simulink model "ASW_PhCurrGen"  (R2023a)
settings: configuration reference "cfg_FastTaskCodeGeneration_v01" (kept outside this file)
undefined symbols (not defined in the file): Cdbl_tiSlwTaskSmpTi, Gu16_psiPermMagFlx_C
settings Model: DataDictionary=dd_foc_dictionary.sldd  EnableAccessToBaseWorkspace=off  Creator=WFYXQ  LastModifiedBy=xiaoqiang.yuan
settings ConfigSetRef: SourceName=cfg_FastTaskCodeGeneration_v01

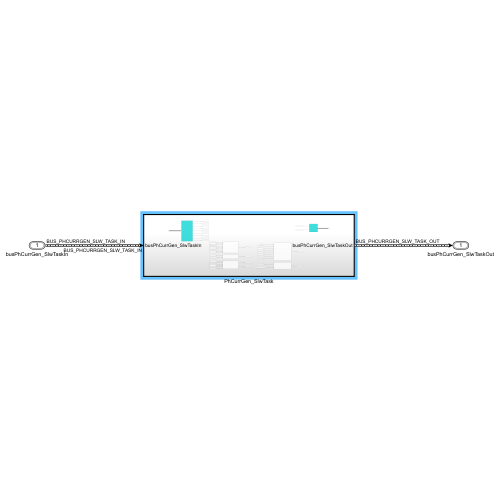
[thumbnail: Simulink's stored preview of the top-level diagram]
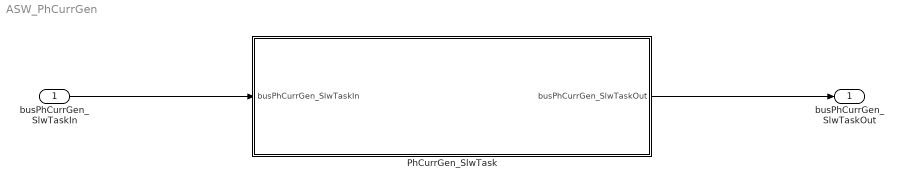
== system ASW_PhCurrGen ==
  busPhCurrGen_SlwTaskIn : Inport  OutDataTypeStr=Bus: BUS_PHCURRGEN_SLW_TASK_IN  SampleTime=round(double(Cdbl_tiSlwTaskSmpTi),4)  BusOutputAsStruct=on
  PhCurrGen_SlwTask : Subsystem  TreatAsAtomicUnit=on  RTWFcnName=PhCurrGen_SlwTask
      settings: RTWSystemCode=Nonreusable function  RTWFcnNameOpts=User specified
  busPhCurrGen_SlwTaskOut : Outport  OutDataTypeStr=Bus: BUS_PHCURRGEN_SLW_TASK_OUT  SampleTime=round(double(Cdbl_tiSlwTaskSmpTi),4)
  wires:
  busPhCurrGen_SlwTaskIn/1 -> PhCurrGen_SlwTask/1(busPhCurrGen_SlwTaskIn)
  PhCurrGen_SlwTask/1(busPhCurrGen_SlwTaskOut) -> busPhCurrGen_SlwTaskOut/1

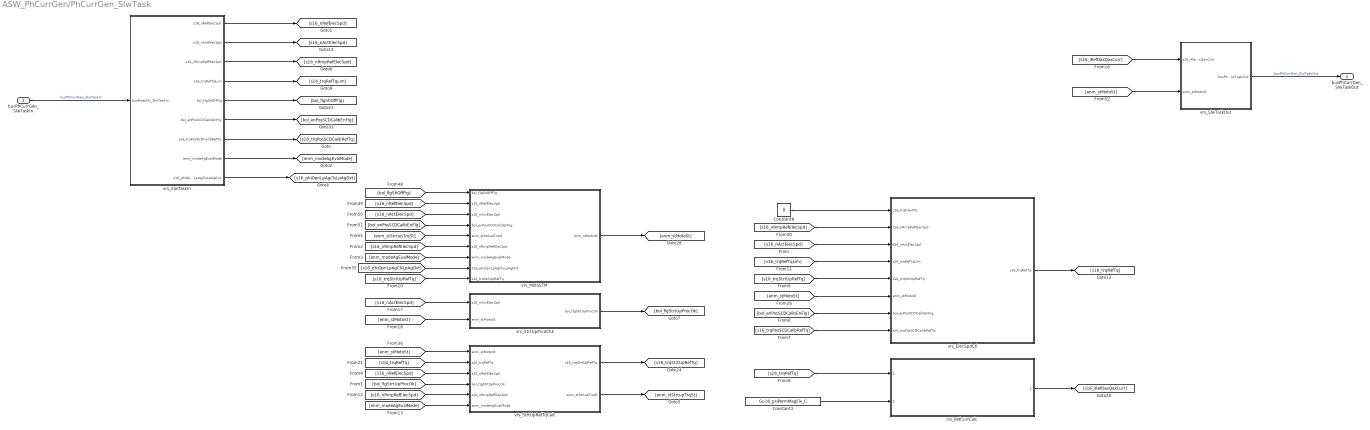
== system ASW_PhCurrGen/PhCurrGen_SlwTask ==
  busPhCurrGen_SlwTaskIn : Inport
  Constant3 : Constant  Value=Gu16_psiPermMagFlx_C
  Constant8 : Constant  Value=0  OutDataTypeStr=dt_Standardize_s16p15b0
  rss_RefCurrCalc : Subsystem  ReferencedSubsystem=rss_RefCurrCalc
  vrs_ElecSpdCtl : Subsystem  Variant=on  VariantControlMode=label  VariantControl=Choice  LabelModeActiveChoice=cstHybrCtrlLbl
  vrs_MotoSTM : Subsystem  Variant=on  VariantControlMode=label  LabelModeActiveChoice=cstHybrCtrlLbl
  vrs_SlwTaskIn : Subsystem  Variant=on  VariantControlMode=label  VariantControl=cstSenlCtrlLbl  LabelModeActiveChoice=cstHybrCtrlLbl
  vrs_SlwTaskOut : Subsystem  Variant=on  VariantControlMode=label  VariantControl=Choice  LabelModeActiveChoice=cstSenlCtrlLbl
  vrs_StrtUpPrcdChk : Subsystem  Variant=on  VariantControlMode=label  LabelModeActiveChoice=cstSenlCtrlLbl
  vrs_StrtUpRefTqCalc : Subsystem  Variant=on  VariantControlMode=label  LabelModeActiveChoice=cstSenlCtrlLbl
  busPhCurrGen_SlwTaskOut : Outport
  wires:
  [s16_trqRefTqLim] -> vrs_ElecSpdCtl/4(s16_trqRefTqLim)
  [s16_iRefDaxQaxCurr] -> vrs_SlwTaskOut/1(s16_iRefDaxQaxCurr)
  Constant8/1 -> vrs_ElecSpdCtl/1(s16_trqFdwdTq)
  vrs_SlwTaskOut/1(busPhCurrGen_SlwTaskOut) -> busPhCurrGen_SlwTaskOut/1  "busPhCurrGen_SlwTaskOut"
  vrs_StrtUpPrcdChk/1(bol_flgStrtUpProcOk) -> [bol_flgStrtUpProcOk]
  [enm_stMotoSt] -> vrs_StrtUpPrcdChk/2(enm_stMotoSt)
  [s16_trqRefTq] -> rss_RefCurrCalc/1
  vrs_ElecSpdCtl/1(s16_trqRefTq) -> [s16_trqRefTq]
  rss_RefCurrCalc/1 -> [s16_iRefDaxQaxCurr]
  [s16_nRmpRefElecSpd] -> vrs_ElecSpdCtl/2(s16_nRmpRefElecSpd)
  [s16_nActElecSpd] -> vrs_StrtUpPrcdChk/1(s16_nActElecSpd)
  [s16_nActElecSpd] -> vrs_ElecSpdCtl/3(s16_nActElecSpd)
  [enm_stMotoSt] -> vrs_ElecSpdCtl/6(enm_stMotoSt)
  [bol_flgShOffFlg] -> vrs_MotoSTM/1(bol_flgShOffFlg)
  [s16_nRefElecSpd] -> vrs_MotoSTM/2(s16_nRefElecSpd)
  [s16_nActElecSpd] -> vrs_MotoSTM/3(s16_nActElecSpd)
  [bol_enPosSCDCalibEnFlg] -> vrs_MotoSTM/4(bol_enPosSCDCalibEnFlg)
  vrs_MotoSTM/1(enm_stMotoSt) -> [enm_stMotoSt]
  [enm_stMotoSt] -> vrs_SlwTaskOut/2(enm_stMotoSt)
  [bol_enPosSCDCalibEnFlg] -> vrs_ElecSpdCtl/7(bol_enPosSCDCalibEnFlg)
  [s16_trqPosSCDCalibRefTq] -> vrs_ElecSpdCtl/8(s16_trqPosSCDCalibRefTq)
  [s16_trqStrtUpRefTq] -> vrs_ElecSpdCtl/5(s16_trqStrtUpRefTq)
  [enm_stMotoSt] -> vrs_StrtUpRefTqCalc/1(enm_stMotoSt)
  [s16_trqRefTq] -> vrs_StrtUpRefTqCalc/2(s16_trqRefTq)
  vrs_StrtUpRefTqCalc/1(s16_trqStrtUpRefTq) -> [s16_trqStrtUpRefTq]
  [s16_nRmpRefElecSpd] -> vrs_MotoSTM/6(s16_nRmpRefElecSpd)
  busPhCurrGen_SlwTaskIn/1 -> vrs_SlwTaskIn/1(busMotoCtl_SlwTaskIn)  "busPhCurrGen_SlwTaskIn"
  vrs_SlwTaskIn/1(s16_nRefElecSpd) -> [s16_nRefElecSpd]
  vrs_SlwTaskIn/2(s16_nActElecSpd) -> [s16_nActElecSpd]
  vrs_SlwTaskIn/3(s16_nRmpRefElecSpd) -> [s16_nRmpRefElecSpd]
  vrs_SlwTaskIn/4(s16_trqRefTqLim) -> [s16_trqRefTqLim]
  vrs_SlwTaskIn/5(bol_flgShOffFlg) -> [bol_flgShOffFlg]
  vrs_SlwTaskIn/6(bol_enPosSCDCalibEnFlg) -> [bol_enPosSCDCalibEnFlg]
  vrs_SlwTaskIn/7(s16_trqPosSCDCalibRefTq) -> [s16_trqPosSCDCalibRefTq]
  vrs_SlwTaskIn/8(enm_modeAgEvalMode) -> [enm_modeAgEvalMode]
  [enm_modeAgEvalMode] -> vrs_MotoSTM/7(enm_modeAgEvalMode)
  Constant3/1 -> rss_RefCurrCalc/2
  [s16_nRefElecSpd] -> vrs_StrtUpRefTqCalc/3(s16_nRefElecSpd)
  vrs_StrtUpRefTqCalc/2(enm_stStrtupTrqSt) -> [enm_stStrtupTrqSt]
  [bol_flgStrtUpProcOk] -> vrs_StrtUpRefTqCalc/4(bol_flgStrtUpProcOk)
  [s16_nRmpRefElecSpd] -> vrs_StrtUpRefTqCalc/5(s16_nRmpRefElecSpd)
  [enm_modeAgEvalMode] -> vrs_StrtUpRefTqCalc/6(enm_modeAgEvalMode)
  [enm_stStrtupTrqSt] -> vrs_MotoSTM/5(enm_stStrtupTrqSt)
  [s16_phiOpnLpAgClsLpAgDvt] -> vrs_MotoSTM/8(s16_phiOpnLpAgClsLpAgDvt)
  [s16_trqStrtUpRefTq] -> vrs_MotoSTM/9(s16_trqStrtUpRefTq)
  vrs_SlwTaskIn/9(s16_phiOpnLpAgClsLpAgDvt) -> [s16_phiOpnLpAgClsLpAgDvt]

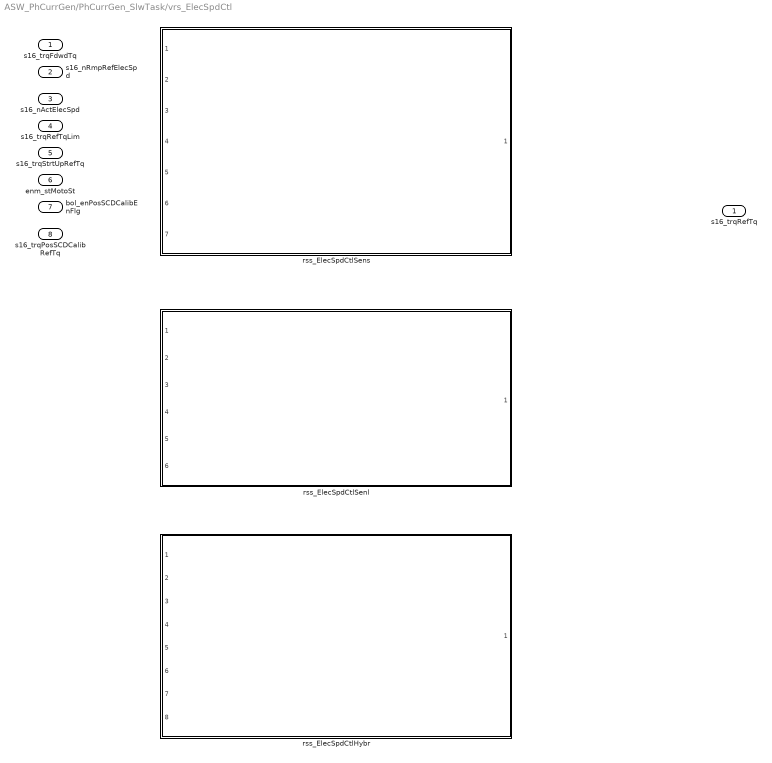
== system ASW_PhCurrGen/PhCurrGen_SlwTask/vrs_ElecSpdCtl ==
  s16_trqFdwdTq : Inport
  s16_nRmpRefElecSpd : Inport  Port=2
  s16_nActElecSpd : Inport  Port=3
  s16_trqRefTqLim : Inport  Port=4
  s16_trqStrtUpRefTq : Inport  Port=5
  enm_stMotoSt : Inport  Port=6
  bol_enPosSCDCalibEnFlg : Inport  Port=7
  s16_trqPosSCDCalibRefTq : Inport  Port=8
  rss_ElecSpdCtlHybr : Subsystem  VariantControl=cstHybrCtrlLbl  ReferencedSubsystem=rss_ElecSpdCtlHybr
  rss_ElecSpdCtlSenl : Subsystem  VariantControl=cstSenlCtrlLbl  ReferencedSubsystem=rss_ElecSpdCtlSenl
  rss_ElecSpdCtlSens : Subsystem  VariantControl=cstSensCtrlLbl  ReferencedSubsystem=rss_ElecSpdCtlSens
  s16_trqRefTq : Outport

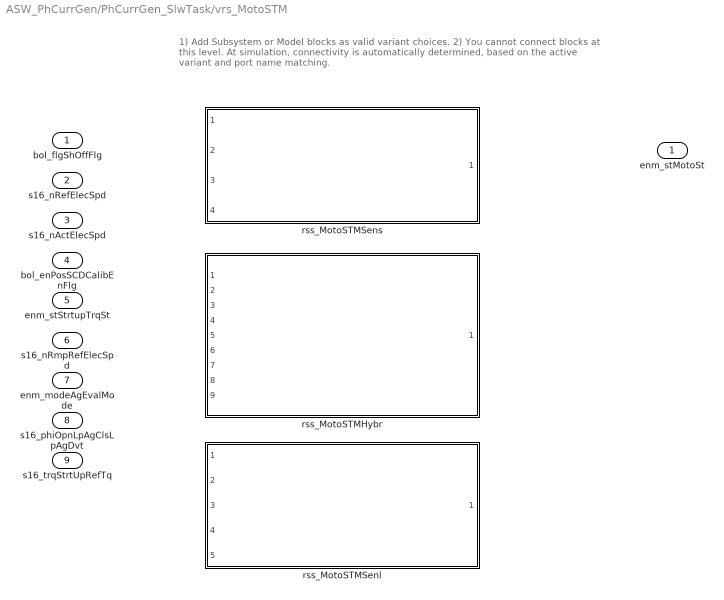
== system ASW_PhCurrGen/PhCurrGen_SlwTask/vrs_MotoSTM ==
  note: 1) Add Subsystem or Model blocks as valid variant choices.
      | 2) You cannot connect blocks at this level. At simulation, connectivity is automatically
      | determined, based on the active variant and port name matching.
  bol_flgShOffFlg : Inport
  s16_nRefElecSpd : Inport  Port=2
  s16_nActElecSpd : Inport  Port=3
  bol_enPosSCDCalibEnFlg : Inport  Port=4
  enm_stStrtupTrqSt : Inport  Port=5
  s16_nRmpRefElecSpd : Inport  Port=6
  enm_modeAgEvalMode : Inport  Port=7
  s16_phiOpnLpAgClsLpAgDvt : Inport  Port=8
  s16_trqStrtUpRefTq : Inport  Port=9
  rss_MotoSTMHybr : Subsystem  VariantControl=cstHybrCtrlLbl  ReferencedSubsystem=rss_MotoSTMHybr
  rss_MotoSTMSenl : Subsystem  VariantControl=cstSenlCtrlLbl  ReferencedSubsystem=rss_MotoSTMSenl
  rss_MotoSTMSens : Subsystem  VariantControl=cstSensCtrlLbl  ReferencedSubsystem=rss_MotoSTMSens
  enm_stMotoSt : Outport

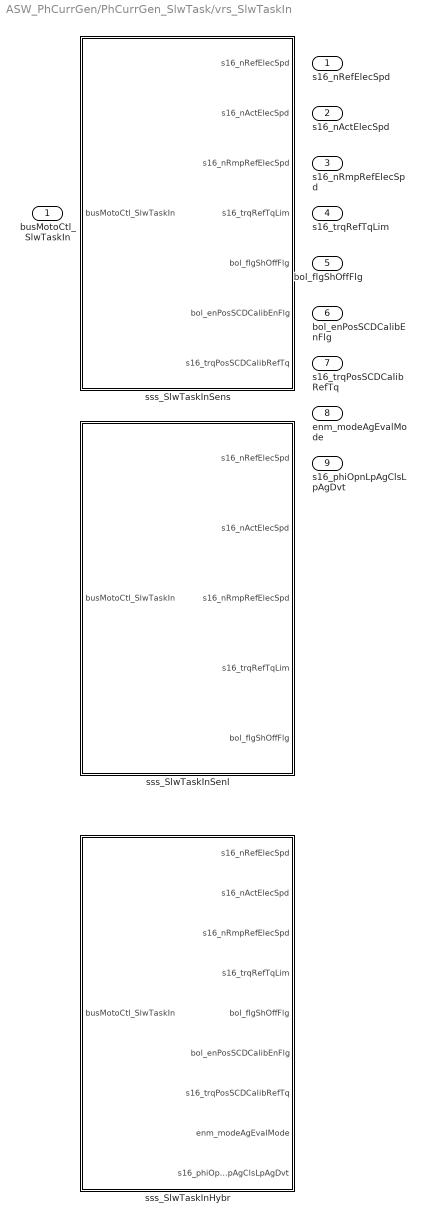
== system ASW_PhCurrGen/PhCurrGen_SlwTask/vrs_SlwTaskIn ==
  busMotoCtl_SlwTaskIn : Inport
  sss_SlwTaskInHybr : Subsystem  VariantControl=cstHybrCtrlLbl
  sss_SlwTaskInSenl : Subsystem  VariantControl=cstSenlCtrlLbl
  sss_SlwTaskInSens : Subsystem  VariantControl=cstSensCtrlLbl
  s16_nRefElecSpd : Outport
  s16_nActElecSpd : Outport  Port=2
  s16_nRmpRefElecSpd : Outport  Port=3
  s16_trqRefTqLim : Outport  Port=4
  bol_flgShOffFlg : Outport  Port=5
  bol_enPosSCDCalibEnFlg : Outport  Port=6
  s16_trqPosSCDCalibRefTq : Outport  Port=7
  enm_modeAgEvalMode : Outport  Port=8
  s16_phiOpnLpAgClsLpAgDvt : Outport  Port=9

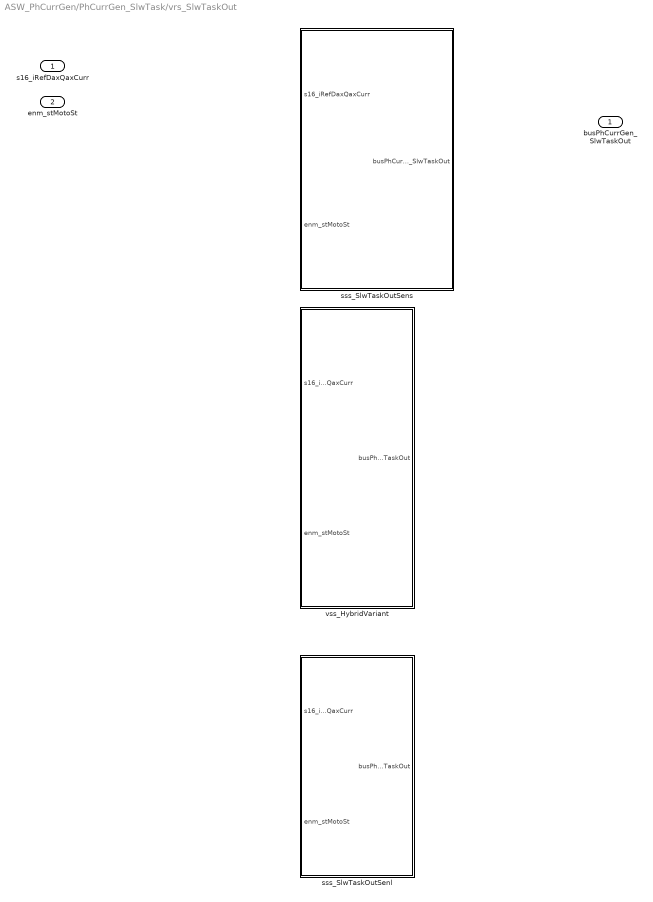
== system ASW_PhCurrGen/PhCurrGen_SlwTask/vrs_SlwTaskOut ==
  s16_iRefDaxQaxCurr : Inport
  enm_stMotoSt : Inport  Port=2
  sss_SlwTaskOutSenl : Subsystem  VariantControl=cstSenlCtrlLbl
  sss_SlwTaskOutSens : Subsystem  VariantControl=cstSensCtrlLbl
  vss_HybridVariant : Subsystem  VariantControl=cstHybrCtrlLbl
  busPhCurrGen_SlwTaskOut : Outport

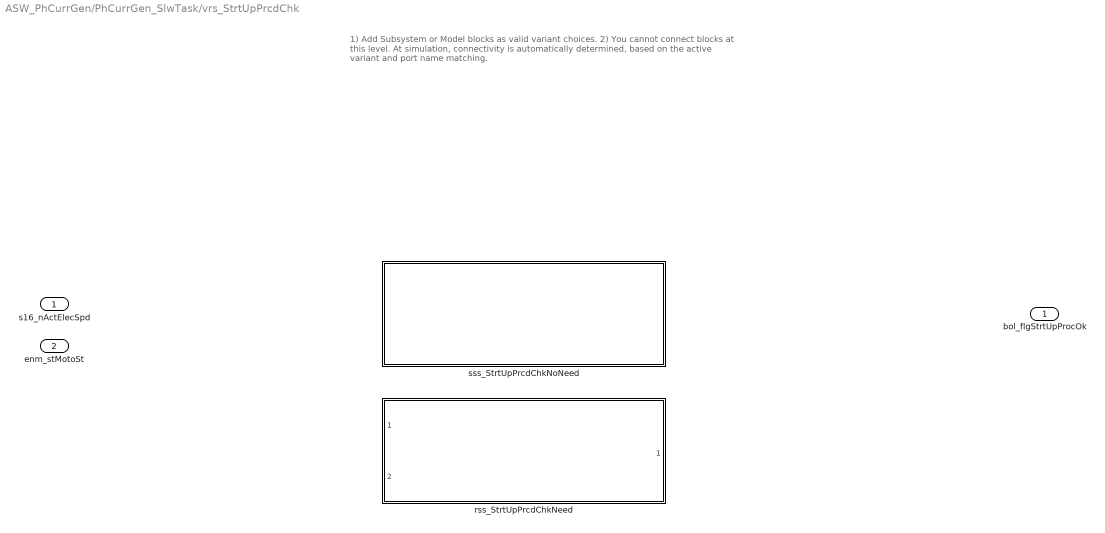
== system ASW_PhCurrGen/PhCurrGen_SlwTask/vrs_StrtUpPrcdChk ==
  note: 1) Add Subsystem or Model blocks as valid variant choices.
      | 2) You cannot connect blocks at this level. At simulation, connectivity is automatically
      | determined, based on the active variant and port name matching.
  s16_nActElecSpd : Inport  PortDimensions=1
  enm_stMotoSt : Inport  Port=2
  rss_StrtUpPrcdChkNeed : Subsystem  VariantControl=cstSenlCtrlLbl  ReferencedSubsystem=rss_StrtUpPrcdChkNeed
  sss_StrtUpPrcdChkNoNeed : Subsystem  VariantControl=cstSensCtrlLbl
  bol_flgStrtUpProcOk : Outport

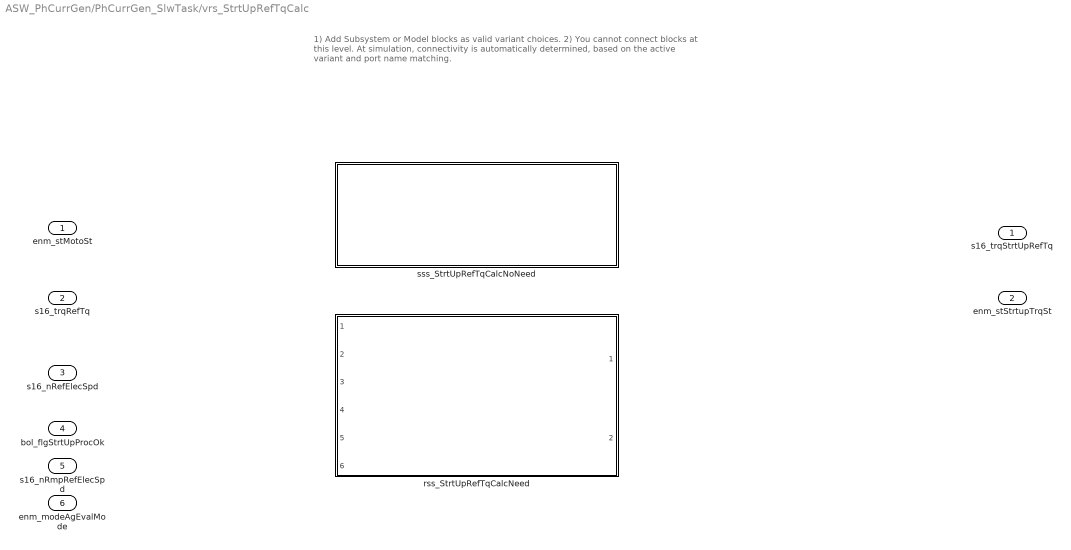
== system ASW_PhCurrGen/PhCurrGen_SlwTask/vrs_StrtUpRefTqCalc ==
  note: 1) Add Subsystem or Model blocks as valid variant choices.
      | 2) You cannot connect blocks at this level. At simulation, connectivity is automatically
      | determined, based on the active variant and port name matching.
  enm_stMotoSt : Inport
  s16_trqRefTq : Inport  Port=2
  s16_nRefElecSpd : Inport  Port=3
  bol_flgStrtUpProcOk : Inport  Port=4
  s16_nRmpRefElecSpd : Inport  Port=5
  enm_modeAgEvalMode : Inport  Port=6
  rss_StrtUpRefTqCalcNeed : Subsystem  VariantControl=cstSenlCtrlLbl  ReferencedSubsystem=rss_StrtUpRefTqCalcNeed
  sss_StrtUpRefTqCalcNoNeed : Subsystem  VariantControl=cstSensCtrlLbl
  s16_trqStrtUpRefTq : Outport
  enm_stStrtupTrqSt : Outport  Port=2

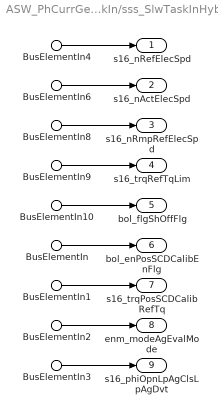
== system ASW_PhCurrGen/PhCurrGen_SlwTask/vrs_SlwTaskIn/sss_SlwTaskInHybr ==
  BusElementIn4 : Inport  PortName=busMotoCtl_SlwTaskIn  Element=s16_nRefElecSpd
  BusElementIn6 : Inport  PortName=busMotoCtl_SlwTaskIn  Element=s16_nActElecSpd
  BusElementIn8 : Inport  PortName=busMotoCtl_SlwTaskIn  Element=s16_nRmpRefElecSpd
  BusElementIn9 : Inport  PortName=busMotoCtl_SlwTaskIn  Element=s16_trqRefTqLim
  BusElementIn10 : Inport  PortName=busMotoCtl_SlwTaskIn  Element=bol_flgShOffFlg
  BusElementIn : Inport  PortName=busMotoCtl_SlwTaskIn  Element=bol_enPosSCDCalibEnFlg
  BusElementIn1 : Inport  PortName=busMotoCtl_SlwTaskIn  Element=s16_trqPosSCDCalibRefTq
  BusElementIn2 : Inport  PortName=busMotoCtl_SlwTaskIn  Element=enm_modeAgEvalMode
  BusElementIn3 : Inport  PortName=busMotoCtl_SlwTaskIn  Element=s16_phiOpnLpAgClsLpAgDvt
  s16_nRefElecSpd : Outport
  s16_nActElecSpd : Outport  Port=2
  s16_nRmpRefElecSpd : Outport  Port=3
  s16_trqRefTqLim : Outport  Port=4
  bol_flgShOffFlg : Outport  Port=5
  bol_enPosSCDCalibEnFlg : Outport  Port=6
  s16_trqPosSCDCalibRefTq : Outport  Port=7
  enm_modeAgEvalMode : Outport  Port=8
  s16_phiOpnLpAgClsLpAgDvt : Outport  Port=9
  wires:
  BusElementIn10/1 -> bol_flgShOffFlg/1
  BusElementIn9/1 -> s16_trqRefTqLim/1
  BusElementIn8/1 -> s16_nRmpRefElecSpd/1
  BusElementIn6/1 -> s16_nActElecSpd/1
  BusElementIn4/1 -> s16_nRefElecSpd/1
  BusElementIn/1 -> bol_enPosSCDCalibEnFlg/1
  BusElementIn1/1 -> s16_trqPosSCDCalibRefTq/1
  BusElementIn2/1 -> enm_modeAgEvalMode/1
  BusElementIn3/1 -> s16_phiOpnLpAgClsLpAgDvt/1

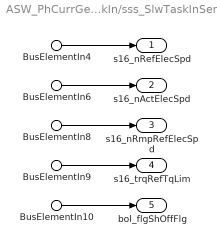
== system ASW_PhCurrGen/PhCurrGen_SlwTask/vrs_SlwTaskIn/sss_SlwTaskInSenl ==
  BusElementIn4 : Inport  PortName=busMotoCtl_SlwTaskIn  Element=s16_nRefElecSpd
  BusElementIn6 : Inport  PortName=busMotoCtl_SlwTaskIn  Element=s16_nActElecSpd
  BusElementIn8 : Inport  PortName=busMotoCtl_SlwTaskIn  Element=s16_nRmpRefElecSpd
  BusElementIn9 : Inport  PortName=busMotoCtl_SlwTaskIn  Element=s16_trqRefTqLim
  BusElementIn10 : Inport  PortName=busMotoCtl_SlwTaskIn  Element=bol_flgShOffFlg
  s16_nRefElecSpd : Outport
  s16_nActElecSpd : Outport  Port=2
  s16_nRmpRefElecSpd : Outport  Port=3
  s16_trqRefTqLim : Outport  Port=4
  bol_flgShOffFlg : Outport  Port=5
  wires:
  BusElementIn4/1 -> s16_nRefElecSpd/1
  BusElementIn6/1 -> s16_nActElecSpd/1
  BusElementIn8/1 -> s16_nRmpRefElecSpd/1
  BusElementIn9/1 -> s16_trqRefTqLim/1
  BusElementIn10/1 -> bol_flgShOffFlg/1

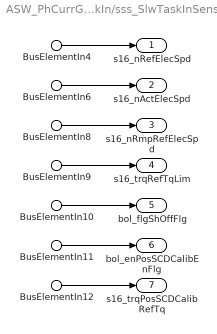
== system ASW_PhCurrGen/PhCurrGen_SlwTask/vrs_SlwTaskIn/sss_SlwTaskInSens ==
  BusElementIn4 : Inport  PortName=busMotoCtl_SlwTaskIn  Element=s16_nRefElecSpd
  BusElementIn6 : Inport  PortName=busMotoCtl_SlwTaskIn  Element=s16_nActElecSpd
  BusElementIn8 : Inport  PortName=busMotoCtl_SlwTaskIn  Element=s16_nRmpRefElecSpd
  BusElementIn9 : Inport  PortName=busMotoCtl_SlwTaskIn  Element=s16_trqRefTqLim
  BusElementIn10 : Inport  PortName=busMotoCtl_SlwTaskIn  Element=bol_flgShOffFlg
  BusElementIn11 : Inport  PortName=busMotoCtl_SlwTaskIn  Element=bol_enPosSCDCalibEnFlg
  BusElementIn12 : Inport  PortName=busMotoCtl_SlwTaskIn  Element=s16_trqPosSCDCalibRefTq
  s16_nRefElecSpd : Outport
  s16_nActElecSpd : Outport  Port=2
  s16_nRmpRefElecSpd : Outport  Port=3
  s16_trqRefTqLim : Outport  Port=4
  bol_flgShOffFlg : Outport  Port=5
  bol_enPosSCDCalibEnFlg : Outport  Port=6
  s16_trqPosSCDCalibRefTq : Outport  Port=7
  wires:
  BusElementIn4/1 -> s16_nRefElecSpd/1
  BusElementIn6/1 -> s16_nActElecSpd/1
  BusElementIn8/1 -> s16_nRmpRefElecSpd/1
  BusElementIn9/1 -> s16_trqRefTqLim/1
  BusElementIn10/1 -> bol_flgShOffFlg/1
  BusElementIn11/1 -> bol_enPosSCDCalibEnFlg/1
  BusElementIn12/1 -> s16_trqPosSCDCalibRefTq/1

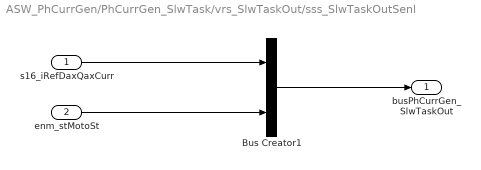
== system ASW_PhCurrGen/PhCurrGen_SlwTask/vrs_SlwTaskOut/sss_SlwTaskOutSenl ==
  s16_iRefDaxQaxCurr : Inport
  enm_stMotoSt : Inport  Port=2
  Bus Creator1 : BusCreator  Inputs=2  OutDataTypeStr=Bus: BUS_PHCURRGEN_SLW_TASK_OUT  NonVirtualBus=on
      settings: InheritFromInputs=off
  busPhCurrGen_SlwTaskOut : Outport
  wires:
  enm_stMotoSt/1 -> Bus Creator1/2
  Bus Creator1/1 -> busPhCurrGen_SlwTaskOut/1
  s16_iRefDaxQaxCurr/1 -> Bus Creator1/1

== system ASW_PhCurrGen/PhCurrGen_SlwTask/vrs_SlwTaskOut/sss_SlwTaskOutSens ==
  s16_iRefDaxQaxCurr : Inport
  enm_stMotoSt : Inport  Port=2
  Bus Creator1 : BusCreator  Inputs=2  OutDataTypeStr=Bus: BUS_PHCURRGEN_SLW_TASK_OUT  NonVirtualBus=on
      settings: InheritFromInputs=off
  busPhCurrGen_SlwTaskOut : Outport
  wires:
  s16_iRefDaxQaxCurr/1 -> Bus Creator1/1
  Bus Creator1/1 -> busPhCurrGen_SlwTaskOut/1
  enm_stMotoSt/1 -> Bus Creator1/2

== system ASW_PhCurrGen/PhCurrGen_SlwTask/vrs_SlwTaskOut/vss_HybridVariant ==
  s16_iRefDaxQaxCurr : Inport
  enm_stMotoSt : Inport  Port=2
  Bus Creator1 : BusCreator  Inputs=2  OutDataTypeStr=Bus: BUS_PHCURRGEN_SLW_TASK_OUT  NonVirtualBus=on
      settings: InheritFromInputs=off
  busPhCurrGen_SlwTaskOut : Outport
  wires:
  s16_iRefDaxQaxCurr/1 -> Bus Creator1/1
  enm_stMotoSt/1 -> Bus Creator1/2
  Bus Creator1/1 -> busPhCurrGen_SlwTaskOut/1

== system ASW_PhCurrGen/PhCurrGen_SlwTask/vrs_StrtUpPrcdChk/sss_StrtUpPrcdChkNoNeed ==

== system ASW_PhCurrGen/PhCurrGen_SlwTask/vrs_StrtUpRefTqCalc/sss_StrtUpRefTqCalcNoNeed ==
